simulink model "InjCrv_PiI1Cor"  (R2016b)
settings: configuration reference "CodeGenConfigSet" (kept outside this file)
values from neighbouring files (symbols this model uses):
  InjCrv_facPiI1APSQCor1EOM0_CUR = Calibration.Parameter    [init_InjCrv_PiI1Cor.m]    (also in init_InjCrv_PiI1Cor_SIL.m = Simulink.Parameter)
  InjCrv_facPiI1APSQCor1EOM0_CURX = Calibration.Parameter    [init_InjCrv_PiI1Cor.m]    (also in init_InjCrv_PiI1Cor_SIL.m = Simulink.Parameter)
  InjCrv_facPiI1APSSOECor1EOM0_CUR = Calibration.Parameter    [init_InjCrv_PiI1Cor.m]    (also in init_InjCrv_PiI1Cor_SIL.m = Simulink.Parameter)
  InjCrv_facPiI1APSSOECor1EOM0_CURX = Calibration.Parameter    [init_InjCrv_PiI1Cor.m]    (also in init_InjCrv_PiI1Cor_SIL.m = Simulink.Parameter)
  InjCrv_facPiI1ATSQCor1EOM0_CUR = Calibration.Parameter    [init_InjCrv_PiI1Cor.m]    (also in init_InjCrv_PiI1Cor_SIL.m = Simulink.Parameter)
  InjCrv_facPiI1ATSQCor1EOM0_CURX = Calibration.Parameter    [init_InjCrv_PiI1Cor.m]    (also in init_InjCrv_PiI1Cor_SIL.m = Simulink.Parameter)
  InjCrv_facPiI1ATSSOECor1EOM0_CUR = Calibration.Parameter    [init_InjCrv_PiI1Cor.m]    (also in init_InjCrv_PiI1Cor_SIL.m = Simulink.Parameter)
  InjCrv_facPiI1ATSSOECor1EOM0_CURX = Calibration.Parameter    [init_InjCrv_PiI1Cor.m]    (also in init_InjCrv_PiI1Cor_SIL.m = Simulink.Parameter)
  InjCrv_facPiI1ETSQCor1EOM0_CUR = Calibration.Parameter    [init_InjCrv_PiI1Cor.m]    (also in init_InjCrv_PiI1Cor_SIL.m = Simulink.Parameter)
  InjCrv_facPiI1ETSQCor1EOM0_CURX = Calibration.Parameter    [init_InjCrv_PiI1Cor.m]    (also in init_InjCrv_PiI1Cor_SIL.m = Simulink.Parameter)
  InjCrv_facPiI1ETSSOECor1EOM0_CUR = Calibration.Parameter    [init_InjCrv_PiI1Cor.m]    (also in init_InjCrv_PiI1Cor_SIL.m = Simulink.Parameter)
  InjCrv_facPiI1ETSSOECor1EOM0_CURX = Calibration.Parameter    [init_InjCrv_PiI1Cor.m]    (also in init_InjCrv_PiI1Cor_SIL.m = Simulink.Parameter)
  InjCrv_phiPiI1APSCor1EOM0_MAP = Calibration.Parameter    [init_InjCrv_PiI1Cor.m]    (also in init_InjCrv_PiI1Cor_SIL.m = Simulink.Parameter)
  InjCrv_phiPiI1APSCor1EOM0_MAPX = Calibration.Parameter    [init_InjCrv_PiI1Cor.m]    (also in init_InjCrv_PiI1Cor_SIL.m = Simulink.Parameter)
  InjCrv_phiPiI1APSCor1EOM0_MAPY = Calibration.Parameter    [init_InjCrv_PiI1Cor.m]    (also in init_InjCrv_PiI1Cor_SIL.m = Simulink.Parameter)
  InjCrv_phiPiI1ATSCor1EOM0_MAP = Calibration.Parameter    [init_InjCrv_PiI1Cor.m]    (also in init_InjCrv_PiI1Cor_SIL.m = Simulink.Parameter)
  InjCrv_phiPiI1ATSCor1EOM0_MAPX = Calibration.Parameter    [init_InjCrv_PiI1Cor.m]    (also in init_InjCrv_PiI1Cor_SIL.m = Simulink.Parameter)
  InjCrv_phiPiI1ATSCor1EOM0_MAPY = Calibration.Parameter    [init_InjCrv_PiI1Cor.m]    (also in init_InjCrv_PiI1Cor_SIL.m = Simulink.Parameter)
  InjCrv_phiPiI1ETSCor1EOM0_MAP = Calibration.Parameter    [init_InjCrv_PiI1Cor.m]    (also in init_InjCrv_PiI1Cor_SIL.m = Simulink.Parameter)
  InjCrv_phiPiI1ETSCor1EOM0_MAPX = Calibration.Parameter    [init_InjCrv_PiI1Cor.m]    (also in init_InjCrv_PiI1Cor_SIL.m = Simulink.Parameter)
  InjCrv_phiPiI1ETSCor1EOM0_MAPY = Calibration.Parameter    [init_InjCrv_PiI1Cor.m]    (also in init_InjCrv_PiI1Cor_SIL.m = Simulink.Parameter)
  InjCrv_qPiI1APSCor1EOM0_MAP = Calibration.Parameter    [init_InjCrv_PiI1Cor.m]    (also in init_InjCrv_PiI1Cor_SIL.m = Simulink.Parameter)
  InjCrv_qPiI1APSCor1EOM0_MAPX = Calibration.Parameter    [init_InjCrv_PiI1Cor.m]    (also in init_InjCrv_PiI1Cor_SIL.m = Simulink.Parameter)
  InjCrv_qPiI1APSCor1EOM0_MAPY = Calibration.Parameter    [init_InjCrv_PiI1Cor.m]    (also in init_InjCrv_PiI1Cor_SIL.m = Simulink.Parameter)
  InjCrv_qPiI1ATSCor1EOM0_MAP = Calibration.Parameter    [init_InjCrv_PiI1Cor.m]    (also in init_InjCrv_PiI1Cor_SIL.m = Simulink.Parameter)
  InjCrv_qPiI1ATSCor1EOM0_MAPX = Calibration.Parameter    [init_InjCrv_PiI1Cor.m]    (also in init_InjCrv_PiI1Cor_SIL.m = Simulink.Parameter)
  InjCrv_qPiI1ATSCor1EOM0_MAPY = Calibration.Parameter    [init_InjCrv_PiI1Cor.m]    (also in init_InjCrv_PiI1Cor_SIL.m = Simulink.Parameter)
  InjCrv_qPiI1ETSCor1EOM0_MAP = Calibration.Parameter    [init_InjCrv_PiI1Cor.m]    (also in init_InjCrv_PiI1Cor_SIL.m = Simulink.Parameter)
  InjCrv_qPiI1ETSCor1EOM0_MAPX = Calibration.Parameter    [init_InjCrv_PiI1Cor.m]    (also in init_InjCrv_PiI1Cor_SIL.m = Simulink.Parameter)
  InjCrv_qPiI1ETSCor1EOM0_MAPY = Calibration.Parameter    [init_InjCrv_PiI1Cor.m]    (also in init_InjCrv_PiI1Cor_SIL.m = Simulink.Parameter)
  InjCrv_tiPiI1APSCor1EOM0_MAP = Calibration.Parameter    [init_InjCrv_PiI1Cor.m]    (also in init_InjCrv_PiI1Cor_SIL.m = Simulink.Parameter)
  InjCrv_tiPiI1APSCor1EOM0_MAPX = Calibration.Parameter    [init_InjCrv_PiI1Cor.m]    (also in init_InjCrv_PiI1Cor_SIL.m = Simulink.Parameter)
  InjCrv_tiPiI1APSCor1EOM0_MAPY = Calibration.Parameter    [init_InjCrv_PiI1Cor.m]    (also in init_InjCrv_PiI1Cor_SIL.m = Simulink.Parameter)
  InjCrv_tiPiI1ATSCor1EOM0_MAP = Calibration.Parameter    [init_InjCrv_PiI1Cor.m]    (also in init_InjCrv_PiI1Cor_SIL.m = Simulink.Parameter)
  InjCrv_tiPiI1ATSCor1EOM0_MAPX = Calibration.Parameter    [init_InjCrv_PiI1Cor.m]    (also in init_InjCrv_PiI1Cor_SIL.m = Simulink.Parameter)
  InjCrv_tiPiI1ATSCor1EOM0_MAPY = Calibration.Parameter    [init_InjCrv_PiI1Cor.m]    (also in init_InjCrv_PiI1Cor_SIL.m = Simulink.Parameter)
  InjCrv_tiPiI1ETSCor1EOM0_MAP = Calibration.Parameter    [init_InjCrv_PiI1Cor.m]    (also in init_InjCrv_PiI1Cor_SIL.m = Simulink.Parameter)
  InjCrv_tiPiI1ETSCor1EOM0_MAPX = Calibration.Parameter    [init_InjCrv_PiI1Cor.m]    (also in init_InjCrv_PiI1Cor_SIL.m = Simulink.Parameter)
  InjCrv_tiPiI1ETSCor1EOM0_MAPY = Calibration.Parameter    [init_InjCrv_PiI1Cor.m]    (also in init_InjCrv_PiI1Cor_SIL.m = Simulink.Parameter)
undefined symbols (not defined in the file or in its folder): HPUn_etaPmp_MAPY
settings Model: Creator=Administrator  LastModifiedBy=mayongchao
settings ConfigSetRef: SourceLocation=Base Workspace

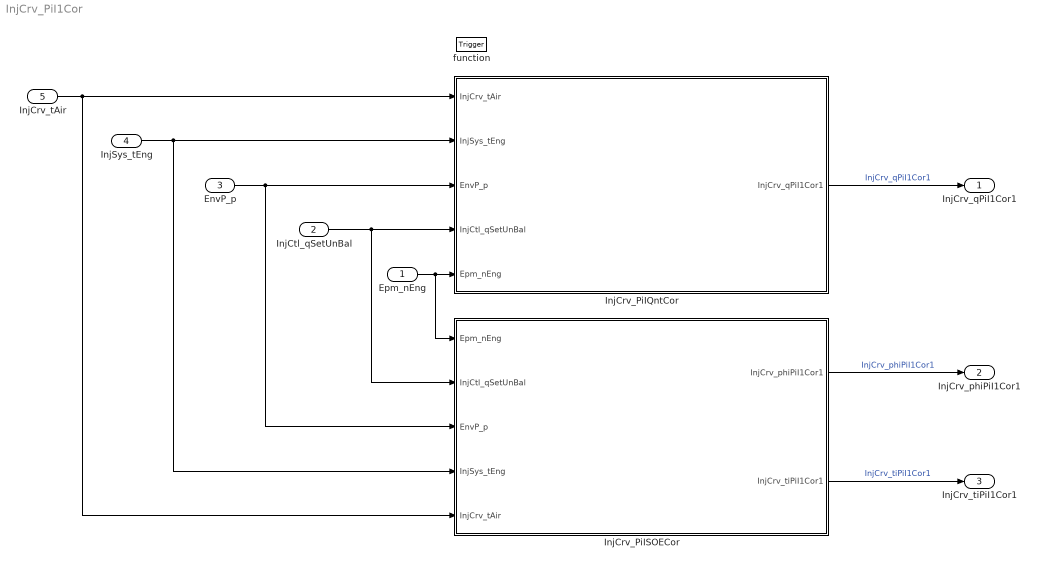
== system InjCrv_PiI1Cor ==
  Epm_nEng : Inport  Tag=rpm  Description=Engine speed  OutMin=0  OutMax=6000  OutDataTypeStr=EngSpeed_rpm
  InjCtl_qSetUnBal : Inport  Tag=mg/hub  Description=Current injection quantity  Port=2  OutMin=-319  OutMax=319  OutDataTypeStr=FuelMass_mg_hub
  EnvP_p : Inport  Tag=kPa  Description=Barometric pressure  Port=3  OutMin=0  OutMax=3276  OutDataTypeStr=AirPressure_kPa
  InjSys_tEng : Inport  Tag=deg  Description=Engine temperature selected for the injection system  Port=4  OutMin=-1000  OutMax=1000  OutDataTypeStr=Temp_deg
  InjCrv_tAir : Inport  Tag=deg  Description=Air temperature for environment corrections  Port=5  OutMin=-50  OutMax=150  OutDataTypeStr=Temp_deg
  function : TriggerPort  TriggerType=function-call  VariantControl=Variant
  InjCrv_PiIQntCor : Subsystem  RTWFcnName=InjCrv_PiIQntCor_Co  RTWFileName=InjCrv_PiIQntCor
      settings: RTWSystemCode=Nonreusable function  RTWFcnNameOpts=User specified  RTWFileNameOpts=User specified
  InjCrv_PiISOECor : Subsystem  RTWFcnName=InjCrv_PiISOECor_Co  RTWFileName=InjCrv_PiISOECor
      settings: RTWSystemCode=Nonreusable function  RTWFcnNameOpts=User specified  RTWFileNameOpts=User specified
  InjCrv_qPiI1Cor1 : Outport  Tag=mg/hub  Description=PiI quantity correction  OutMin=-319  OutMax=319  OutDataTypeStr=FuelMass_mg_hub
  InjCrv_phiPiI1Cor1 : Outport  Tag=CA  Description=PiI1 start of energizing correction(phi)  Port=2  OutMin=-719  OutMax=719  OutDataTypeStr=Angle_CA
  InjCrv_tiPiI1Cor1 : Outport  Tag=us  Description=PiI1 start of energizing correction(ti)  Port=3  OutMin=-13107  OutMax=13106  OutDataTypeStr=InjTime_us
  wires:
  InjCrv_PiIQntCor/1(InjCrv_qPiI1Cor1) -> InjCrv_qPiI1Cor1/1  "InjCrv_qPiI1Cor1"
  InjCrv_PiISOECor/1(InjCrv_phiPiI1Cor1) -> InjCrv_phiPiI1Cor1/1  "InjCrv_phiPiI1Cor1"
  InjCrv_PiISOECor/2(InjCrv_tiPiI1Cor1) -> InjCrv_tiPiI1Cor1/1  "InjCrv_tiPiI1Cor1"
  Epm_nEng/1 -> InjCrv_PiISOECor/1(Epm_nEng), InjCrv_PiIQntCor/5(Epm_nEng)
  InjCrv_tAir/1 -> InjCrv_PiIQntCor/1(InjCrv_tAir), InjCrv_PiISOECor/5(InjCrv_tAir)
  InjSys_tEng/1 -> InjCrv_PiISOECor/4(InjSys_tEng), InjCrv_PiIQntCor/2(InjSys_tEng)
  EnvP_p/1 -> InjCrv_PiIQntCor/3(EnvP_p), InjCrv_PiISOECor/3(EnvP_p)
  InjCtl_qSetUnBal/1 -> InjCrv_PiIQntCor/4(InjCtl_qSetUnBal), InjCrv_PiISOECor/2(InjCtl_qSetUnBal)

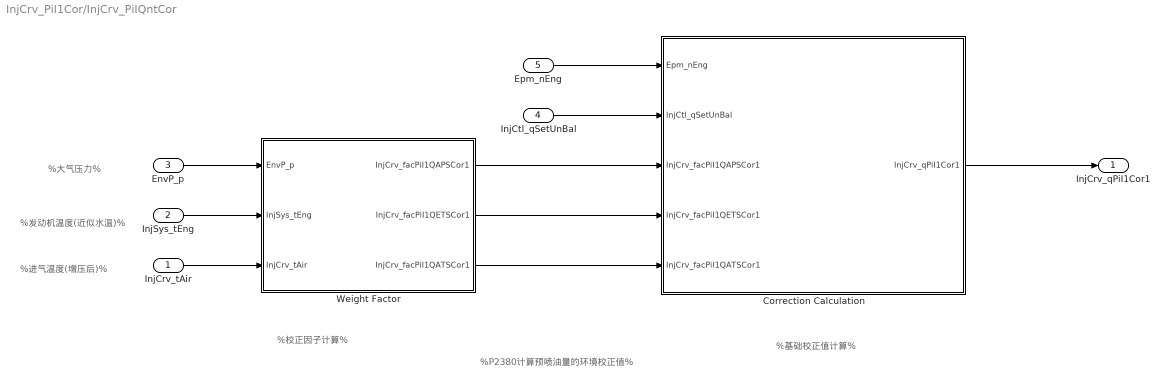
== system InjCrv_PiI1Cor/InjCrv_PiIQntCor ==
  note: %P2380计算预喷油量的环境校正值%
  note: %进气温度(增压后)%
  note: %发动机温度(近似水温)%
  note: %大气压力%
  note: %校正因子计算%
  note: %基础校正值计算%
  InjCrv_tAir : Inport
  InjSys_tEng : Inport  Port=2
  EnvP_p : Inport  Port=3
  InjCtl_qSetUnBal : Inport  Port=4
  Epm_nEng : Inport  Port=5
  Correction Calculation : Subsystem  RequirementInfo={'other' 'InjCrv_PiI_requirements.doc' '@Simulink_requirement_item_10' 'true' '预喷油量环境校正值计算' '' } %GIDa_56448458_d2a4_412d_85d8_cf76f2bb3a8d
  Weight Factor : Subsystem  RequirementInfo={'other' 'InjCrv_PiI_requirements.doc' '@Simulink_requirement_item_9' 'true' '预喷油量校正因子计算' '' } %GIDa_982227b5_8c17_4b18_84bc_fea40f3ff8d7
  InjCrv_qPiI1Cor1 : Outport
  wires:
  Correction Calculation/1(InjCrv_qPiI1Cor1) -> InjCrv_qPiI1Cor1/1
  Weight Factor/3(InjCrv_facPiI1QATSCor1) -> Correction Calculation/5(InjCrv_facPiI1QATSCor1)
  Weight Factor/2(InjCrv_facPiI1QETSCor1) -> Correction Calculation/4(InjCrv_facPiI1QETSCor1)
  Weight Factor/1(InjCrv_facPiI1QAPSCor1) -> Correction Calculation/3(InjCrv_facPiI1QAPSCor1)
  InjCtl_qSetUnBal/1 -> Correction Calculation/2(InjCtl_qSetUnBal)
  Epm_nEng/1 -> Correction Calculation/1(Epm_nEng)
  InjCrv_tAir/1 -> Weight Factor/3(InjCrv_tAir)
  InjSys_tEng/1 -> Weight Factor/2(InjSys_tEng)
  EnvP_p/1 -> Weight Factor/1(EnvP_p)

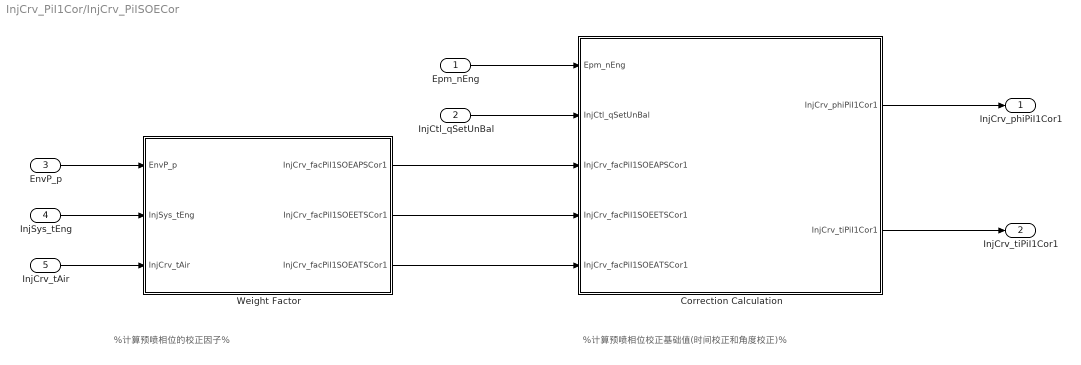
== system InjCrv_PiI1Cor/InjCrv_PiISOECor ==
  note: %计算预喷相位的校正因子%
  note: %计算预喷相位校正基础值(时间校正和角度校正)%
  Epm_nEng : Inport
  InjCtl_qSetUnBal : Inport  Port=2
  EnvP_p : Inport  Port=3
  InjSys_tEng : Inport  Port=4
  InjCrv_tAir : Inport  Port=5
  Correction Calculation : Subsystem  RequirementInfo={'other' 'InjCrv_PiI_requirements.doc' '@Simulink_requirement_item_16' 'true' '预喷相位校正值计算' '' } %GIDa_7c3028f7_9900_445e_be56_6b5e274f5338
  Weight Factor : Subsystem  RequirementInfo={'other' 'InjCrv_PiI_requirements.doc' '@Simulink_requirement_item_15' 'true' '预喷相位校正因子计算' '' } %GIDa_48cf1669_5401_4188_9b6a_cc07e0c26cf4
  InjCrv_phiPiI1Cor1 : Outport
  InjCrv_tiPiI1Cor1 : Outport  Port=2
  wires:
  Correction Calculation/2(InjCrv_tiPiI1Cor1) -> InjCrv_tiPiI1Cor1/1
  InjCtl_qSetUnBal/1 -> Correction Calculation/2(InjCtl_qSetUnBal)
  Epm_nEng/1 -> Correction Calculation/1(Epm_nEng)
  InjCrv_tAir/1 -> Weight Factor/3(InjCrv_tAir)
  InjSys_tEng/1 -> Weight Factor/2(InjSys_tEng)
  EnvP_p/1 -> Weight Factor/1(EnvP_p)
  Correction Calculation/1(InjCrv_phiPiI1Cor1) -> InjCrv_phiPiI1Cor1/1
  Weight Factor/3(InjCrv_facPiI1SOEATSCor1) -> Correction Calculation/5(InjCrv_facPiI1SOEATSCor1)
  Weight Factor/2(InjCrv_facPiI1SOEETSCor1) -> Correction Calculation/4(InjCrv_facPiI1SOEETSCor1)
  Weight Factor/1(InjCrv_facPiI1SOEAPSCor1) -> Correction Calculation/3(InjCrv_facPiI1SOEAPSCor1)

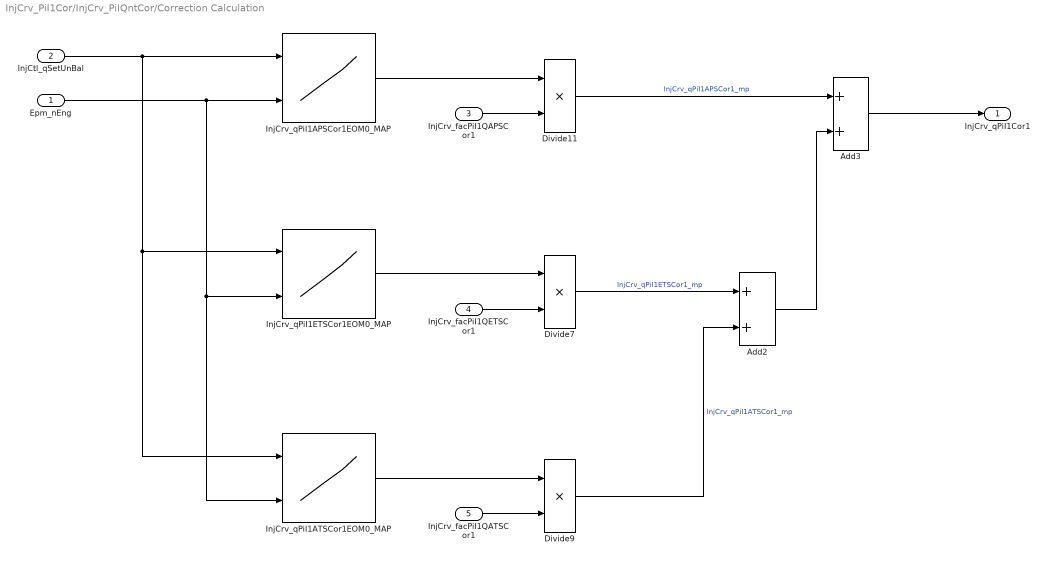
== system InjCrv_PiI1Cor/InjCrv_PiIQntCor/Correction Calculation ==
  Epm_nEng : Inport
  InjCtl_qSetUnBal : Inport  Port=2
  InjCrv_facPiI1QAPSCor1 : Inport  Port=3
  InjCrv_facPiI1QETSCor1 : Inport  Port=4
  InjCrv_facPiI1QATSCor1 : Inport  Port=5
  Add2 : Sum  InputSameDT=on
  Add3 : Sum  InputSameDT=on
  Divide11 : Product  Inputs=**  OutDataTypeStr=FuelMass_mg_hub
  Divide7 : Product  Inputs=**  OutDataTypeStr=FuelMass_mg_hub
  Divide9 : Product  Inputs=**  OutDataTypeStr=FuelMass_mg_hub
  InjCrv_qPiI1APSCor1EOM0_MAP : Lookup_n-D  BreakpointsForDimension1=InjCrv_qPiI1APSCor1EOM0_MAPY  BreakpointsForDimension2=InjCrv_qPiI1APSCor1EOM0_MAPX  IndexSearchMethod=Linear search  BeginIndexSearchUsingPreviousIndexResult=on  Table=InjCrv_qPiI1APSCor1EOM0_MAP  ExtrapMethod=Clip  UseLastTableValue=on  InternalRulePriority=Speed  OutDataTypeStr=Inherit: Inherit via back propagation  SaturateOnIntegerOverflow=on
  InjCrv_qPiI1ATSCor1EOM0_MAP : Lookup_n-D  BreakpointsForDimension1=InjCrv_qPiI1ATSCor1EOM0_MAPY  BreakpointsForDimension2=InjCrv_qPiI1ATSCor1EOM0_MAPX  IndexSearchMethod=Linear search  BeginIndexSearchUsingPreviousIndexResult=on  Table=InjCrv_qPiI1ATSCor1EOM0_MAP  ExtrapMethod=Clip  UseLastTableValue=on  InternalRulePriority=Speed  OutDataTypeStr=Inherit: Inherit via back propagation  SaturateOnIntegerOverflow=on
  InjCrv_qPiI1ETSCor1EOM0_MAP : Lookup_n-D  BreakpointsForDimension1=InjCrv_qPiI1ETSCor1EOM0_MAPY  BreakpointsForDimension2=InjCrv_qPiI1ETSCor1EOM0_MAPX  IndexSearchMethod=Linear search  BeginIndexSearchUsingPreviousIndexResult=on  Table=InjCrv_qPiI1ETSCor1EOM0_MAP  ExtrapMethod=Clip  UseLastTableValue=on  InternalRulePriority=Speed  OutDataTypeStr=Inherit: Inherit via back propagation  SaturateOnIntegerOverflow=on
  InjCrv_qPiI1Cor1 : Outport
  wires:
  Add3/1 -> InjCrv_qPiI1Cor1/1
  Divide9/1 -> Add2/2  "InjCrv_qPiI1ATSCor1_mp"
  InjCrv_facPiI1QATSCor1/1 -> Divide9/2
  InjCrv_qPiI1ATSCor1EOM0_MAP/1 -> Divide9/1
  Add2/1 -> Add3/2
  Divide7/1 -> Add2/1  "InjCrv_qPiI1ETSCor1_mp"
  InjCrv_facPiI1QETSCor1/1 -> Divide7/2
  InjCrv_qPiI1ETSCor1EOM0_MAP/1 -> Divide7/1
  Divide11/1 -> Add3/1  "InjCrv_qPiI1APSCor1_mp"
  InjCrv_facPiI1QAPSCor1/1 -> Divide11/2
  InjCrv_qPiI1APSCor1EOM0_MAP/1 -> Divide11/1
  InjCtl_qSetUnBal/1 -> InjCrv_qPiI1APSCor1EOM0_MAP/1, InjCrv_qPiI1ATSCor1EOM0_MAP/1, InjCrv_qPiI1ETSCor1EOM0_MAP/1
  Epm_nEng/1 -> InjCrv_qPiI1APSCor1EOM0_MAP/2, InjCrv_qPiI1ATSCor1EOM0_MAP/2, InjCrv_qPiI1ETSCor1EOM0_MAP/2

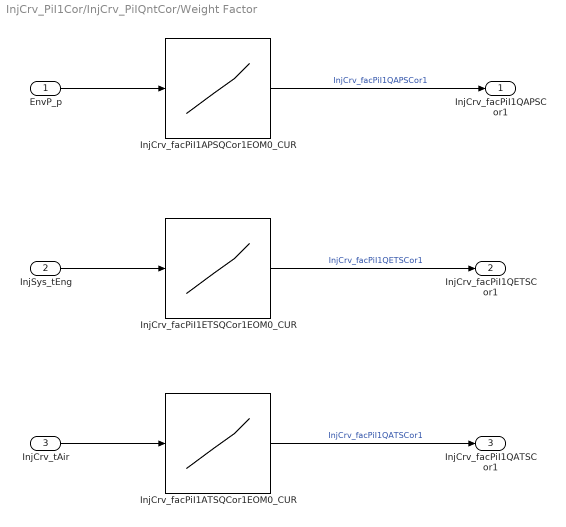
== system InjCrv_PiI1Cor/InjCrv_PiIQntCor/Weight Factor ==
  EnvP_p : Inport
  InjSys_tEng : Inport  Port=2
  InjCrv_tAir : Inport  Port=3
  InjCrv_facPiI1APSQCor1EOM0_CUR : Lookup_n-D  NumberOfTableDimensions=1  BreakpointsForDimension1=InjCrv_facPiI1APSQCor1EOM0_CURX  BreakpointsForDimension2=HPUn_etaPmp_MAPY  IndexSearchMethod=Linear search  BeginIndexSearchUsingPreviousIndexResult=on  Table=InjCrv_facPiI1APSQCor1EOM0_CUR  ExtrapMethod=Clip  UseLastTableValue=on  InternalRulePriority=Speed  OutDataTypeStr=Inherit: Inherit via back propagation  SaturateOnIntegerOverflow=on
  InjCrv_facPiI1ATSQCor1EOM0_CUR : Lookup_n-D  NumberOfTableDimensions=1  BreakpointsForDimension1=InjCrv_facPiI1ATSQCor1EOM0_CURX  BreakpointsForDimension2=HPUn_etaPmp_MAPY  IndexSearchMethod=Linear search  BeginIndexSearchUsingPreviousIndexResult=on  Table=InjCrv_facPiI1ATSQCor1EOM0_CUR  ExtrapMethod=Clip  UseLastTableValue=on  InternalRulePriority=Speed  OutDataTypeStr=Inherit: Inherit via back propagation  SaturateOnIntegerOverflow=on
  InjCrv_facPiI1ETSQCor1EOM0_CUR : Lookup_n-D  NumberOfTableDimensions=1  BreakpointsForDimension1=InjCrv_facPiI1ETSQCor1EOM0_CURX  BreakpointsForDimension2=HPUn_etaPmp_MAPY  IndexSearchMethod=Linear search  BeginIndexSearchUsingPreviousIndexResult=on  Table=InjCrv_facPiI1ETSQCor1EOM0_CUR  ExtrapMethod=Clip  UseLastTableValue=on  InternalRulePriority=Speed  OutDataTypeStr=Inherit: Inherit via back propagation  SaturateOnIntegerOverflow=on
  InjCrv_facPiI1QAPSCor1 : Outport
  InjCrv_facPiI1QETSCor1 : Outport  Port=2
  InjCrv_facPiI1QATSCor1 : Outport  Port=3
  wires:
  EnvP_p/1 -> InjCrv_facPiI1APSQCor1EOM0_CUR/1
  InjCrv_facPiI1ATSQCor1EOM0_CUR/1 -> InjCrv_facPiI1QATSCor1/1  "InjCrv_facPiI1QATSCor1"
  InjCrv_facPiI1ETSQCor1EOM0_CUR/1 -> InjCrv_facPiI1QETSCor1/1  "InjCrv_facPiI1QETSCor1"
  InjCrv_facPiI1APSQCor1EOM0_CUR/1 -> InjCrv_facPiI1QAPSCor1/1  "InjCrv_facPiI1QAPSCor1"
  InjCrv_tAir/1 -> InjCrv_facPiI1ATSQCor1EOM0_CUR/1
  InjSys_tEng/1 -> InjCrv_facPiI1ETSQCor1EOM0_CUR/1

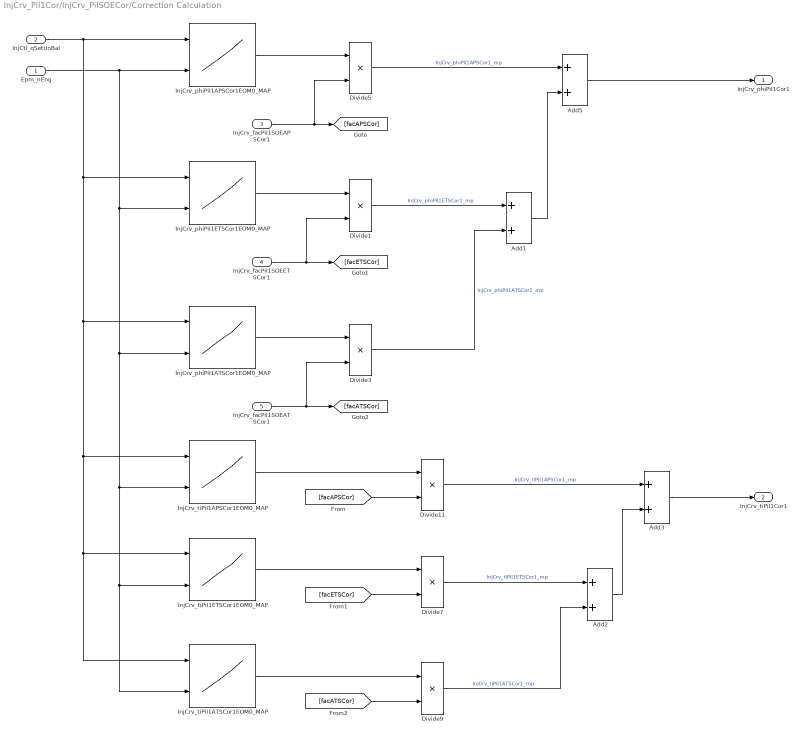
== system InjCrv_PiI1Cor/InjCrv_PiISOECor/Correction Calculation ==
  Epm_nEng : Inport
  InjCtl_qSetUnBal : Inport  Port=2
  InjCrv_facPiI1SOEAPSCor1 : Inport  Port=3
  InjCrv_facPiI1SOEETSCor1 : Inport  Port=4
  InjCrv_facPiI1SOEATSCor1 : Inport  Port=5
  Add{1..3,5} (4 alike) : Sum  InputSameDT=on
  Divide1 : Product  Inputs=**  OutDataTypeStr=Angle_CA
  Divide11 : Product  Inputs=**  OutDataTypeStr=InjTime_us
  Divide3 : Product  Inputs=**  OutDataTypeStr=Angle_CA
  Divide5 : Product  Inputs=**  OutDataTypeStr=Angle_CA
  Divide7 : Product  Inputs=**  OutDataTypeStr=InjTime_us
  Divide9 : Product  Inputs=**  OutDataTypeStr=InjTime_us
  InjCrv_phiPiI1APSCor1EOM0_MAP : Lookup_n-D  BreakpointsForDimension1=InjCrv_phiPiI1APSCor1EOM0_MAPY  BreakpointsForDimension2=InjCrv_phiPiI1APSCor1EOM0_MAPX  IndexSearchMethod=Linear search  BeginIndexSearchUsingPreviousIndexResult=on  Table=InjCrv_phiPiI1APSCor1EOM0_MAP  ExtrapMethod=Clip  UseLastTableValue=on  InternalRulePriority=Speed  OutDataTypeStr=Inherit: Inherit via back propagation  SaturateOnIntegerOverflow=on
  InjCrv_phiPiI1ATSCor1EOM0_MAP : Lookup_n-D  BreakpointsForDimension1=InjCrv_phiPiI1ATSCor1EOM0_MAPY  BreakpointsForDimension2=InjCrv_phiPiI1ATSCor1EOM0_MAPX  IndexSearchMethod=Linear search  BeginIndexSearchUsingPreviousIndexResult=on  Table=InjCrv_phiPiI1ATSCor1EOM0_MAP  ExtrapMethod=Clip  UseLastTableValue=on  InternalRulePriority=Speed  OutDataTypeStr=Inherit: Inherit via back propagation  SaturateOnIntegerOverflow=on
  InjCrv_phiPiI1ETSCor1EOM0_MAP : Lookup_n-D  BreakpointsForDimension1=InjCrv_phiPiI1ETSCor1EOM0_MAPY  BreakpointsForDimension2=InjCrv_phiPiI1ETSCor1EOM0_MAPX  IndexSearchMethod=Linear search  BeginIndexSearchUsingPreviousIndexResult=on  Table=InjCrv_phiPiI1ETSCor1EOM0_MAP  ExtrapMethod=Clip  UseLastTableValue=on  InternalRulePriority=Speed  OutDataTypeStr=Inherit: Inherit via back propagation  SaturateOnIntegerOverflow=on
  InjCrv_tiPiI1APSCor1EOM0_MAP : Lookup_n-D  BreakpointsForDimension1=InjCrv_tiPiI1APSCor1EOM0_MAPY  BreakpointsForDimension2=InjCrv_tiPiI1APSCor1EOM0_MAPX  IndexSearchMethod=Linear search  BeginIndexSearchUsingPreviousIndexResult=on  Table=InjCrv_tiPiI1APSCor1EOM0_MAP  ExtrapMethod=Clip  UseLastTableValue=on  InternalRulePriority=Speed  OutDataTypeStr=Inherit: Inherit via back propagation  SaturateOnIntegerOverflow=on
  InjCrv_tiPiI1ATSCor1EOM0_MAP : Lookup_n-D  BreakpointsForDimension1=InjCrv_tiPiI1ATSCor1EOM0_MAPY  BreakpointsForDimension2=InjCrv_tiPiI1ATSCor1EOM0_MAPX  IndexSearchMethod=Linear search  BeginIndexSearchUsingPreviousIndexResult=on  Table=InjCrv_tiPiI1ATSCor1EOM0_MAP  ExtrapMethod=Clip  UseLastTableValue=on  InternalRulePriority=Speed  OutDataTypeStr=Inherit: Inherit via back propagation  SaturateOnIntegerOverflow=on
  InjCrv_tiPiI1ETSCor1EOM0_MAP : Lookup_n-D  BreakpointsForDimension1=InjCrv_tiPiI1ETSCor1EOM0_MAPY  BreakpointsForDimension2=InjCrv_tiPiI1ETSCor1EOM0_MAPX  IndexSearchMethod=Linear search  BeginIndexSearchUsingPreviousIndexResult=on  Table=InjCrv_tiPiI1ETSCor1EOM0_MAP  ExtrapMethod=Clip  UseLastTableValue=on  InternalRulePriority=Speed  OutDataTypeStr=Inherit: Inherit via back propagation  SaturateOnIntegerOverflow=on
  InjCrv_phiPiI1Cor1 : Outport
  InjCrv_tiPiI1Cor1 : Outport  Port=2
  wires:
  [facATSCor] -> Divide9/2
  [facETSCor] -> Divide7/2
  [facAPSCor] -> Divide11/2
  Add3/1 -> InjCrv_tiPiI1Cor1/1
  Divide9/1 -> Add2/2  "InjCrv_tiPiI1ATSCor1_mp"
  InjCrv_tiPiI1ATSCor1EOM0_MAP/1 -> Divide9/1
  Add2/1 -> Add3/2
  Divide7/1 -> Add2/1  "InjCrv_tiPiI1ETSCor1_mp"
  InjCrv_tiPiI1ETSCor1EOM0_MAP/1 -> Divide7/1
  Divide11/1 -> Add3/1  "InjCrv_tiPiI1APSCor1_mp"
  InjCrv_tiPiI1APSCor1EOM0_MAP/1 -> Divide11/1
  Add5/1 -> InjCrv_phiPiI1Cor1/1
  Divide3/1 -> Add1/2  "InjCrv_phiPiI1ATSCor1_mp"
  InjCrv_facPiI1SOEATSCor1/1 -> Divide3/2, [facATSCor]
  InjCrv_phiPiI1ATSCor1EOM0_MAP/1 -> Divide3/1
  Add1/1 -> Add5/2
  Divide1/1 -> Add1/1  "InjCrv_phiPiI1ETSCor1_mp"
  InjCrv_facPiI1SOEETSCor1/1 -> [facETSCor], Divide1/2
  InjCrv_phiPiI1ETSCor1EOM0_MAP/1 -> Divide1/1
  Divide5/1 -> Add5/1  "InjCrv_phiPiI1APSCor1_mp"
  InjCrv_facPiI1SOEAPSCor1/1 -> [facAPSCor], Divide5/2
  InjCtl_qSetUnBal/1 -> InjCrv_tiPiI1ATSCor1EOM0_MAP/1, InjCrv_tiPiI1ETSCor1EOM0_MAP/1, InjCrv_tiPiI1APSCor1EOM0_MAP/1, InjCrv_phiPiI1ATSCor1EOM0_MAP/1, InjCrv_phiPiI1ETSCor1EOM0_MAP/1, InjCrv_phiPiI1APSCor1EOM0_MAP/1
  Epm_nEng/1 -> InjCrv_phiPiI1APSCor1EOM0_MAP/2, InjCrv_tiPiI1ATSCor1EOM0_MAP/2, InjCrv_tiPiI1ETSCor1EOM0_MAP/2, InjCrv_tiPiI1APSCor1EOM0_MAP/2, InjCrv_phiPiI1ATSCor1EOM0_MAP/2, InjCrv_phiPiI1ETSCor1EOM0_MAP/2
  InjCrv_phiPiI1APSCor1EOM0_MAP/1 -> Divide5/1

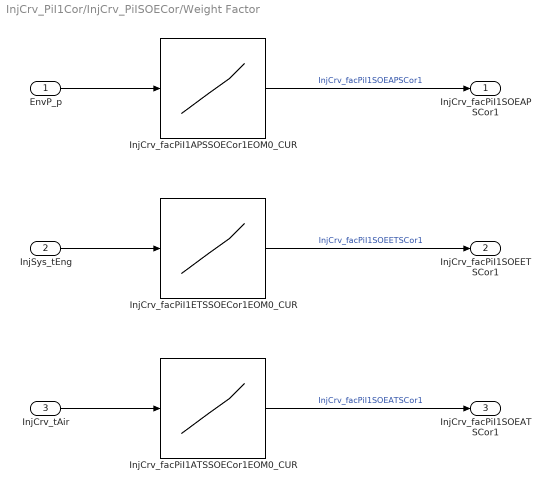
== system InjCrv_PiI1Cor/InjCrv_PiISOECor/Weight Factor ==
  EnvP_p : Inport
  InjSys_tEng : Inport  Port=2
  InjCrv_tAir : Inport  Port=3
  InjCrv_facPiI1APSSOECor1EOM0_CUR : Lookup_n-D  NumberOfTableDimensions=1  BreakpointsForDimension1=InjCrv_facPiI1APSSOECor1EOM0_CURX  BreakpointsForDimension2=HPUn_etaPmp_MAPY  IndexSearchMethod=Linear search  BeginIndexSearchUsingPreviousIndexResult=on  Table=InjCrv_facPiI1APSSOECor1EOM0_CUR  ExtrapMethod=Clip  UseLastTableValue=on  InternalRulePriority=Speed  OutDataTypeStr=Inherit: Inherit via back propagation  SaturateOnIntegerOverflow=on
  InjCrv_facPiI1ATSSOECor1EOM0_CUR : Lookup_n-D  NumberOfTableDimensions=1  BreakpointsForDimension1=InjCrv_facPiI1ATSSOECor1EOM0_CURX  BreakpointsForDimension2=HPUn_etaPmp_MAPY  IndexSearchMethod=Linear search  BeginIndexSearchUsingPreviousIndexResult=on  Table=InjCrv_facPiI1ATSSOECor1EOM0_CUR  ExtrapMethod=Clip  UseLastTableValue=on  InternalRulePriority=Speed  OutDataTypeStr=Inherit: Inherit via back propagation  SaturateOnIntegerOverflow=on
  InjCrv_facPiI1ETSSOECor1EOM0_CUR : Lookup_n-D  NumberOfTableDimensions=1  BreakpointsForDimension1=InjCrv_facPiI1ETSSOECor1EOM0_CURX  BreakpointsForDimension2=HPUn_etaPmp_MAPY  IndexSearchMethod=Linear search  BeginIndexSearchUsingPreviousIndexResult=on  Table=InjCrv_facPiI1ETSSOECor1EOM0_CUR  ExtrapMethod=Clip  UseLastTableValue=on  InternalRulePriority=Speed  OutDataTypeStr=Inherit: Inherit via back propagation  SaturateOnIntegerOverflow=on
  InjCrv_facPiI1SOEAPSCor1 : Outport
  InjCrv_facPiI1SOEETSCor1 : Outport  Port=2
  InjCrv_facPiI1SOEATSCor1 : Outport  Port=3
  wires:
  InjCrv_facPiI1ATSSOECor1EOM0_CUR/1 -> InjCrv_facPiI1SOEATSCor1/1  "InjCrv_facPiI1SOEATSCor1"
  InjCrv_tAir/1 -> InjCrv_facPiI1ATSSOECor1EOM0_CUR/1
  InjCrv_facPiI1ETSSOECor1EOM0_CUR/1 -> InjCrv_facPiI1SOEETSCor1/1  "InjCrv_facPiI1SOEETSCor1"
  InjSys_tEng/1 -> InjCrv_facPiI1ETSSOECor1EOM0_CUR/1
  InjCrv_facPiI1APSSOECor1EOM0_CUR/1 -> InjCrv_facPiI1SOEAPSCor1/1  "InjCrv_facPiI1SOEAPSCor1"
  EnvP_p/1 -> InjCrv_facPiI1APSSOECor1EOM0_CUR/1
